simulink model "balance_region_schedule"  (R2021a)
settings: Solver=FixedStepDiscrete  StartTime=0.0  StopTime=5000  RelTol=1e-6
model workspace (MAT data in the model file):
  Ts = 10
  a_amp = 1.1
  a_capacity = 100
  a_initial_available = 10
  b_amp = 1.1
  b_capacity = 100
  b_initial_available = 100
  consumer_size = 1000
  low_space_ratio = 0.8
  move = 0.004
  op_finish_duration = 60
  store_limit = 15
  write_qps = 0
undefined symbols (not defined in the file or in its folder): DiscIntNeverNeededParam
libraries: pingcap x5, simulink x2
settings Model: OrderedModelArguments=off  Creator=tongjian  LastModifiedBy=tongjian

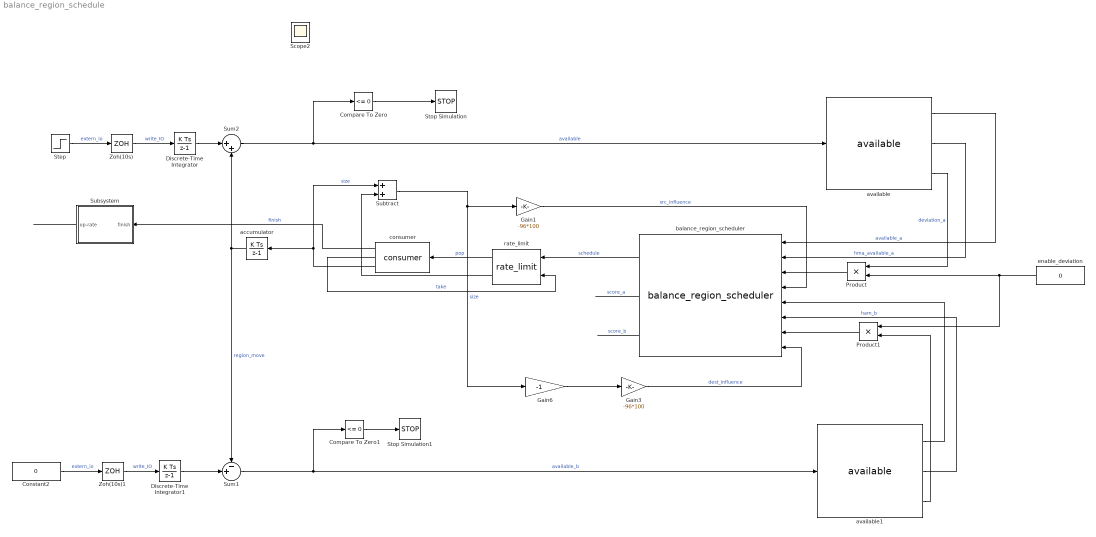
== system balance_region_schedule ==
  Compare To Zero : simulink/Logic and Bit Operations/Compare To Zero  relop=<=  OutDataTypeStr=boolean
  Compare To Zero1 : simulink/Logic and Bit Operations/Compare To Zero  relop=<=  OutDataTypeStr=boolean
  Constant2 : Constant  Value=0
  Discrete-Time Integrator : DiscreteIntegrator  gainval=1  InitialCondition=a_initial_available  SampleTime=Ts  ICPrevOutput=DiscIntNeverNeededParam  ICPrevScaledInput=DiscIntNeverNeededParam
  Discrete-Time Integrator1 : DiscreteIntegrator  gainval=1  InitialCondition=b_initial_available  SampleTime=Ts  ICPrevOutput=DiscIntNeverNeededParam  ICPrevScaledInput=DiscIntNeverNeededParam
  Gain1 : Gain  Gain=-96*100
  Gain3 : Gain  Gain=-96*100
  Gain6 : Gain  Gain=-1
  Product : Product
  Product1 : Product
  Step : Step  Time=40*60  After=write_qps  SampleTime=0
  Stop Simulation : Stop
  Stop Simulation1 : Stop
  Subsystem : Subsystem
  Subtract : Sum
  Sum1 : Sum  Inputs=-+|
  Sum2 : Sum  Inputs=|++
  Zoh(10s) : ZeroOrderHold  Description=Zoh(10s)  SampleTime=Ts
  Zoh(10s)1 : ZeroOrderHold  Description=Zoh(10s)  SampleTime=Ts
  accumulator : DiscreteIntegrator  gainval=96*10/(1024*a_amp*op_finish_duration)  SampleTime=-1  ICPrevOutput=DiscIntNeverNeededParam  ICPrevScaledInput=DiscIntNeverNeededParam
  available : pingcap/available  g_Ts=Ts  g_hma_nums_deviation_0=hma_nums_deviation_0  g_hma_dens_deviation_0=hma_dens_deviation_0  g_hma_nums_deviation_1=hma_nums_deviation_1  g_hma_dens_deviation_1=hma_dens_deviation_0  g_hma_nums_deviation_2=hma_nums_deviation_2  g_hma_dens_deviation_2=hma_dens_deviation_0  g_hma_nums_avg_0=hma_nums_avg_0  g_hma_dens_avg_0=hma_dens_avg_0  g_hma_nums_avg_1=hma_nums_avg_0  g_hma_dens_avg_1=hma_dens_avg_0  g_hma_nums_avg_2=hma_nums_avg_0  g_hma_dens_avg_2=hma_dens_avg_0  g_initial=a_initial_available
  available1 : pingcap/available  g_Ts=Ts  g_hma_nums_deviation_0=hma_nums_deviation_0  g_hma_dens_deviation_0=hma_dens_deviation_0  g_hma_nums_deviation_1=hma_nums_deviation_1  g_hma_dens_deviation_1=hma_dens_deviation_0  g_hma_nums_deviation_2=hma_nums_deviation_2  g_hma_dens_deviation_2=hma_dens_deviation_0  g_hma_nums_avg_0=hma_nums_avg_0  g_hma_dens_avg_0=hma_dens_avg_0  g_hma_nums_avg_1=hma_nums_avg_0  g_hma_dens_avg_1=hma_dens_avg_0  g_hma_nums_avg_2=hma_nums_avg_0  g_hma_dens_avg_2=hma_dens_avg_0  g_initial=b_initial_available
  "balance_region_scheduler " : pingcap/balance_region_scheduler   g_a_capacity=a_capacity  g_b_capacity=b_capacity  g_a_amp=a_amp  g_b_amp=b_amp  g_low_space_ratio=0.8
      link override "balance_region_scheduler ": SystemSampleTime=-1
  consumer : pingcap/consumer  g_consumer_size=consumer_size  g_consumer_duration=op_finish_duration  g_Ts=0.1
  enable_deviation : Constant  Value=0
  rate_limit : pingcap/rate_limit  g_store_limit=store_limit  g_Ts=0.1
  Scope2 : Scope
  wires:
  Zoh(10s)/1 -> Discrete-Time Integrator/1  "write_IO"
  Step/1 -> Zoh(10s)/1  "extern_io"
  Constant2/1 -> Zoh(10s)1/1  "extern_io"
  Zoh(10s)1/1 -> Discrete-Time Integrator1/1  "write_IO"
  Gain6/1 -> Gain3/1
  Compare To Zero/1 -> Stop Simulation/1
  Discrete-Time Integrator/1 -> Sum2/1
  Sum2/1 -> Compare To Zero/1, available/1  "available"
  accumulator/1 -> Sum1/1, Sum2/2  "region_move"
  available/1 -> "balance_region_scheduler "/1  "available_a"
  available/2 -> "balance_region_scheduler "/2  "hma_available_a"
  available1/1 -> "balance_region_scheduler "/5
  available1/2 -> "balance_region_scheduler "/6  "ham_b"
  Gain3/1 -> "balance_region_scheduler "/8  "dest_influence"
  "balance_region_scheduler "/1 -> rate_limit/1  "schedule"
  rate_limit/1 -> consumer/1  "pop"
  rate_limit/2 -> Subtract/2
  "balance_region_scheduler "/2 -> ?  "score_a"
  "balance_region_scheduler "/3 -> ?  "score_b"
  Discrete-Time Integrator1/1 -> Sum1/2
  Sum1/1 -> Compare To Zero1/1, available1/1  "available_b"
  consumer/2 -> rate_limit/2  "take"
  consumer/3 -> accumulator/1, Subtract/1  "size"
  Subtract/1 -> Gain1/1, Gain6/1  "size"
  Product/1 -> "balance_region_scheduler "/3
  available/3 -> Product/1  "deviation_a"
  enable_deviation/1 -> Product/2, Product1/1
  Product1/1 -> "balance_region_scheduler "/7
  available1/3 -> Product1/2
  Compare To Zero1/1 -> Stop Simulation1/1
  Gain1/1 -> "balance_region_scheduler "/4  "src_influence"
  consumer/1 -> Subsystem/1(finish)  "finish"
  Subsystem/1(op-rate) -> ?

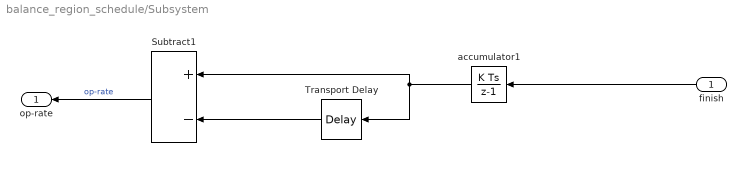
== system balance_region_schedule/Subsystem ==
  finish : Inport
  Subtract1 : Sum  Inputs=+-
  Transport Delay : TransportDelay  DelayTime=60  FixedBuffer=on
  accumulator1 : DiscreteIntegrator  gainval=Ts  SampleTime=-1  ICPrevOutput=DiscIntNeverNeededParam  ICPrevScaledInput=DiscIntNeverNeededParam
  op-rate : Outport
  wires:
  Subtract1/1 -> op-rate/1  "op-rate"
  Transport Delay/1 -> Subtract1/2
  finish/1 -> accumulator1/1
  accumulator1/1 -> Transport Delay/1, Subtract1/1
